simulink model "torque_controller"  (R2018b)
settings: Solver=VariableStepAuto  StartTime=0.0  StopTime=1000  RelTol=1e-3
values from neighbouring files (symbols this model uses):
  ADAMS_cwd = 'C:\Users\Daniel\Documents\GitKraken\DVA439-bicycle-balancing\simulations\simulink'    [Nonlinear_Torque_12km.m]
  ADAMS_exec = ''    [Nonlinear_Torque_12km.m]
  ADAMS_host = 'LAPTOP-BA4FLL9Q'    [Nonlinear_Torque_12km.m]
  ADAMS_init = ''    [Nonlinear_Torque_12km.m]
  ADAMS_inputs = 'TorqueMotor.var_motor_torque!V_In!FrameDisturbance'    [Nonlinear_Torque_12km.m]
  ADAMS_outputs = 'LeanAng_In!SteerAngle!V_Out!Dist!DriftAngle'    [Nonlinear_Torque_12km.m]
  ADAMS_prefix = 'Nonlinear_Torque_12km'    [Nonlinear_Torque_12km.m]
  ADAMS_static = 'no'    [Nonlinear_Torque_12km.m]
  ADAMS_sysdir = 'C:\PROGRA~1\MSC~1.SOF\ADAMSS~1\2018_1\'    [Nonlinear_Torque_12km.m]
libraries: simulink_extras x3, dspsrcs4 x2, simulink x2
settings Model: Creator=Daniel  LastModifiedBy=Daniel
settings SolverCC: AlgebraicLoopSolver=LineSearch

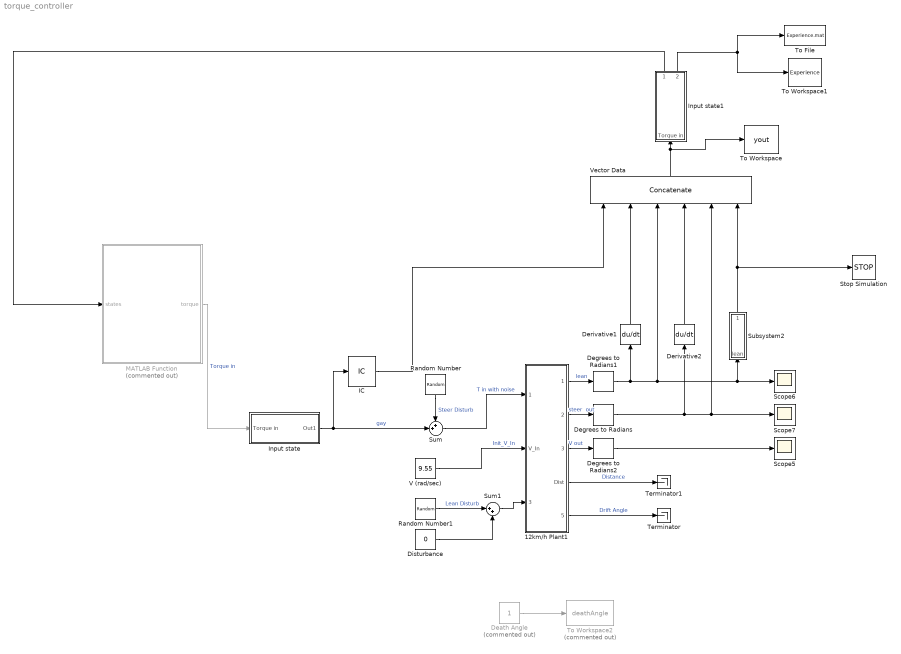
== system torque_controller ==
  12km/h Plant1 : Subsystem
  Death Angle : Constant  Commented=on  SampleTime=-1
  Degrees to Radians : simulink_extras/Transformations/Degrees to Radians
  Degrees to Radians1 : simulink_extras/Transformations/Degrees to Radians
  Degrees to Radians2 : simulink_extras/Transformations/Degrees to Radians
  Derivative1 : Derivative
  Derivative2 : Derivative
  Disturbance : Constant  Value=0
  IC : InitialCondition  Value=0
  Input state : Subsystem
  Input state1 : Subsystem
  MATLAB Function : MATLAB Function  Commented=on  TreatAsAtomicUnit=on
  Random Number : RandomNumber  Variance=0.1  SampleTime=0.1
  Random Number1 : RandomNumber  Variance=0.1  SampleTime=0.1
  Scope5 : Scope
  Scope6 : Scope
  Scope7 : Scope
  Stop Simulation : Stop
  Subsystem2 : Subsystem
  Sum : Sum  Inputs=++|
  Sum1 : Sum  Inputs=|++
  Terminator : Terminator
  Terminator1 : Terminator
  To File : ToFile  Filename=Experience.mat
  To Workspace : ToWorkspace  VariableName=yout  SampleTime=-1
      settings: Save2DSignal=2-D array (concatenate along first dimension)
  To Workspace1 : ToWorkspace  VariableName=Experience  SampleTime=-1
      settings: Decimation=2
  To Workspace2 : ToWorkspace  Commented=on  VariableName=deathAngle  SampleTime=-1
      settings: MaxDataPoints=1
  V (rad/sec) : Constant  Value=9.55
  Vector Data : Concatenate  NumInputs=6
  wires:
  Random Number1/1 -> Sum1/1  "Lean Disturb"
  Disturbance/1 -> Sum1/2
  12km/h Plant1/5(DriftAngle) -> Terminator/1  "Drift Angle"
  Random Number/1 -> Sum/1  "Steer Disturb"
  12km/h Plant1/4("Dist      ") -> Terminator1/1  "Distance"
  Degrees to Radians/1 -> Derivative2/1, Vector Data/5, Scope7/1
  V (rad/sec)/1 -> 12km/h Plant1/2("V_In                        ")  "Init_V_In"
  12km/h Plant1/2(SteerAngle) -> Degrees to Radians/1  "steer  out"
  Sum1/1 -> 12km/h Plant1/3("FrameDisturbance            ")
  12km/h Plant1/3("V_Out     ") -> Degrees to Radians2/1  "V out"
  Sum/1 -> 12km/h Plant1/1(TorqueMotor.var_motor_torque)  "T in with noise"
  Degrees to Radians2/1 -> Scope5/1
  Derivative1/1 -> Vector Data/2
  Derivative2/1 -> Vector Data/4
  Vector Data/1 -> To Workspace/1, Input state1/1(Torque in)
  IC/1 -> Vector Data/1
  Subsystem2/1(dead lean) -> Stop Simulation/1, Vector Data/6
  Death Angle/1 -> To Workspace2/1
  MATLAB Function/1(torque) -> Input state/1(Torque in)  "Torque in"
  Degrees to Radians1/1 -> Derivative1/1, Vector Data/3, Subsystem2/1(lean), Scope6/1
  12km/h Plant1/1(LeanAng_In) -> Degrees to Radians1/1  "lean"
  Input state/1(Out1) -> IC/1, Sum/2  "gay"
  Input state1/1(Out1) -> MATLAB Function/1(states)
  Input state1/2(Out2) -> To File/1, To Workspace1/1

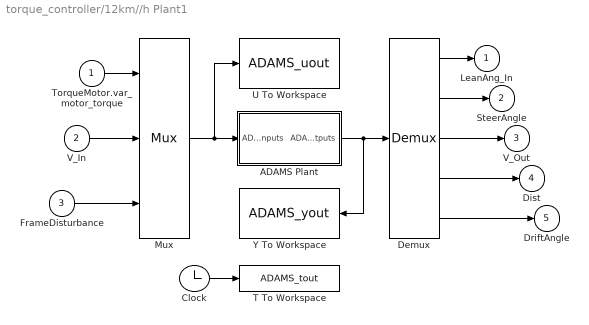
== system torque_controller/12km//h Plant1 ==
  TorqueMotor.var_motor_torque : Inport
  "V_In                        " : Inport  Port=2
  "FrameDisturbance            " : Inport  Port=3
  ADAMS Plant : Subsystem  LoadFcn=|  InitFcn=clear mex  mask(Adams Plant){exevie=ADAMS_sysdir, nam_in=ADAMS_inputs, namout=ADAMS_outputs, nampre=ADAMS_prefix, outfil=ADAMS_prefix, exesol=ADAMS_exec, stat=ADAMS_static, inicmd=[ADAMS_init], exetyp=C++, comtyp=PIPE(DDE), workdir=ADAMS_cwd, ada_host=ADAMS_host, modani=batch, modsim=discrete, dft=no, simulink_lead_cosim=yes, pin_interp_order=0, pout_extrap_order=0, pin_extrap_order=0, pout_interp_order=0, dt_out=0.005, o_rate=1, more=off}
      | %check based on dialog box setting for when setting by popup menu                                             
      | if exist('ADAMS_solver_type')                                                                                 
      |   if strcmp(ADAMS_solver_type,'C++')                                                                          
      |     set_param(gcb,'exetyp','C++');                                                                            
      |   else                                                                                                        
      |     set_param(gcb,'exetyp','Fortran');                                                                        
      |   end                                                                                                         
      | else                                                                                                          
      |   set_param(gcb,'exetyp','C++');                                                                              
      | end                                                                                                           
      | %set the mode if using acar_solver                                                                            
      | %REQUIRED HERE BECAUSE BELOW CAUSES MDLTERMINATE TO BE CALLED 2 TIMES IN MIDDLE OF SIMULATION WHEN SET IN MASK
      |                                                                                                               
      | %enable the direct feedthrough, sim mode, anim mode parameters by default                                     
      |                                                                                                               
      | if exist('set_some_params_states')                                                                            
      |                                                                                                               
      |   set_some_params_states({'dft','modsim','modani'},{'on','on','on'},'MaskEnables',gcb)                        
      |   %turn on direct feedthrough option                                                                          
      |   set_some_params_states({'dft'},{'on'},'MaskVisibilities',gcb)                                               
      |                                                                                                               
      |  end                                                                                                          
      |                                                                                                               
      |                                                                                                               
      | if exist('ADAMS_exec')                                                                                        
      |   if and(strcmp(get_param(gcb,'exesol'),'ADAMS_exec'),strcmp(ADAMS_exec,'acar_solver'))                       
      |     %set the sim mode to discrete -- only supported mode                                                      
      |     set_param(gcb,'modsim','discrete')                                                                        
      |      %turn off direct feedthrough option                                                                      
      |      set_some_params_states({'dft'},{'off'},'MaskVisibilities',gcb)                                           
      |     %set the animation mode to batch -- only supported mode                                                   
      |     set_param(gcb,'modani','batch')                                                                           
      |     %disable the direct feedthrough, sim mode, anim mode parameters                                           
      |     set_some_params_states({'modsim','modani'},{'off','off'},'MaskEnables',gcb)                               
      |   end                                                                                                         
      | end
      mask prompts: exevie "Adams install directory"; nam_in "Adams View input names"; namout "Adams View output names"; nampre "Adams model file prefix"; outfil "Output files prefix (opt.: if blank - no output)"; exesol "User executable (opt.: if blank - use standard)"; stat "Initial static simulation flag"; inicmd "Initialization commands"; exetyp "Adams Solver type"; comtyp "Interprocess option"; workdir "Adams working directory"; ada_host "Adams host"; modani "Animation mode"; modsim "Simulation mode"; dft "Direct feedthrough"; simulink_lead_cosim "Discrete Computational Order - Simulink Leads Adams"; pin_interp_order "Plant input interpolation order"; pout_extrap_order "Plant output extrapolation order"; pin_extrap_order "Plant input extrapolation order"; pout_interp_order "Plant output interpolation order"; dt_out "Communication interval"; o_rate "Number of communications per output step"; more "More parameters"
      mask help: Simulate any Adams plant model either in Adams Solver form (.adm file) or in Adams View form (.cmd file)
      settings: OpenFcn=|
      | open_system(gcb,'mask')
      | if not(exist('set_some_params_states'))
      | 
      | warning('The script "set_some_params_states.m" cannot be found in the MATLAB PATH.  Cannot update the ADAMS Plant S-Function parameters.')
      | 
      | warning('Recommended action(optional):  run the Adams Controls .m file first to help choose the correct settings in the Adams S-Function block.')
      | 
      | end
      mask Help:
      | <html>
      | This S-Function represents the non-linear Adams Plant with the inputs sent to the Adams model <br>
      |  and the outputs generated by the Adams model.  See the Adams Controls documentation for more <br>
      | information.  This plant uses the following variables:<br>
      | <br>
      | <b>ADAMS_sysdir  :</b> Adams installation directory<br>
      | <b>ADAMS_inputs  :</b> Input variables View names vector<br>
      | <b>ADAMS_outputs :</b> Outputs variables View names vector<br>
      | <b>ADAMS_prefix  : </b>ADAMS model files prefix (.adm, .cmd); also doubles as output files prefix<br>
      | <b>ADAMS_exec :</b> Adams Solver user library or keyword (e.g., acar_solver)<br>
      | <b>ADAMS_static :</b> yes|no - initial static before Co-simulation(discrete)/Function Evaluation(continuous)<br>
      | <b>ADAMS_init :</b>Initialization commands (i.e., Adams View or Solver commands, depending on setting for Animation mode)<br>
      | <b>ADAMS_cwd : </b> Current working directory (for TCP/IP)<br>
      | <b>ADAMS_host : </b>Name of Adams server host (for TCP/IP)<br>
      | <b>ADAMS_mode :</b> Linear or non-linear (i.e., co-sim, function eval)<br>
      | <b>ADAMS_solver_type :</b>Fortran or C++ (used to set popup menu when first loaded) <br>
      | 
      | 
      | <br>
      | The following settings can be chosen:<br>
      | <br>
      | <b>Adams Solver type:</b>  Fortran or C++ (will also set ADAMS_solver_type)<br>
      | <b>Interprocess option:</b> Pipe(DDE) or TCP/IP; TCP/IP can allow different machines run Adams and MATLAB<br>
      | <b>Animation mode:</b> batch (Solver, uses .adm) or interactive (View, uses .cmd)<br>
      | <b>Simulation mode:</b> discrete (Co-simulation) or continuous (Function Evaluation)<br>
      | <b>Discrete Computational Order - Simulink Lead Adams:</b> for discrete mode, chooses if Simulink leads the integration (yes) or lags (no);<br> if set to "no", can remove algebraic loop<br>
      | <b>Plant input interpolation order:</b> 0 = zero-order hold; 1 = linear (discrete mode only, where Simulink leads)<br>
      | <b>Plant output extrapolation order:</b> 0 = zero-order hold;1 = linear(discrete mode only, where Simulink leads)<br>
      | <b>Plant input extrapolation order:</b> 0 = zero-order hold; 1 = linear (discrete mode only, where Adams leads)<br>
      | <b>Plant output interpolation order:</b> 0 = zero-order hold;1 = linear(discrete mode only, where Adams leads)<br>
      | <b>Direct feedthrough:</b> yes|no - yes = Input directly effect output(continuous mode-only)<br>
      | <b>Communication interval:</b> Time step at which Co-simulation exchange information (e.g.,0.005); also controls <br>output for continuous mode (Function Evaluation)<br>
      | <b>Number of communications per output step: </b>Sets Adams output rate (.res, .req, .gra) integer value (default: 1)<br>
      | </html>
      mask Callback exesol:
      | if exist('set_some_params_states')
      | %enable the direct feedthrough, sim mode, anim mode parameters
      | set_some_params_states({'dft','modsim','modani'},{'on','on','on'},'MaskEnables',gcb)
      | %turn on direct feedthrough option
      | set_some_params_states({'dft'},{'on'},'MaskVisibilities',gcb)
      | end
      | 
      | if exist('ADAMS_exec')
      |   if and(strcmp(get_param(gcb,'exesol'),'ADAMS_exec'),strcmp(ADAMS_exec,'acar_solver'))
      |     %set the sim mode to discrete -- only supported mode
      |     %REMOVED:  BELOW CAUSES MDLTERMINATE TO BE CALLED 2 TIMES IN MIDDLE OF SIMULATION
      |     %Now in LoadFcn callback
      |     %set_param(gcb,'modsim','discrete')
      |      %turn off direct feedthrough option
      |     set_some_params_states({'dft'},{'off'},'MaskVisibilities',gcb)
      |     %set the animation mode to batch -- only supported mode
      |     %REMOVED:  BELOW CAUSES MDLTERMINATE TO BE CALLED 2 TIMES IN MIDDLE OF SIMULATION
      |     %Now in LoadFcn callback
      |     %set_param(gcb,'modani','batch')
      |     %disable the direct feedthrough, sim mode, anim mode parameters
      |     set_some_params_states({'modsim','modani'},{'off','off'},'MaskEnables',gcb)
      |   end
      | end
      mask TypeOptions exetyp: Fortran | C++
      mask Callback exetyp:
      | if strcmp(get_param(gcb,'exetyp'),'C++')
      |     ADAMS_solver_type='C++';
      | else
      |     ADAMS_solver_type='Fortran';
      | end
      mask TypeOptions comtyp: PIPE(DDE) | TCP/IP
      mask Callback comtyp:
      | if exist('set_some_params_states')
      | if strcmp(get_param(gcb,'comtyp'),'PIPE(DDE)')
      |     %turn off cwd, host options
      |     set_some_params_states({'ada_host','workdir'},{'off','off'},'MaskVisibilities',gcb)
      | else%if strcmp(get_param(gcb,'modsim'),'TCP/IP')
      |     %turn on cwd, host options
      |     set_some_params_states({'ada_host','workdir'},{'on','on'},'MaskVisibilities',gcb)
      | end
      | end
      mask TypeOptions modani: batch | interactive
      mask TypeOptions modsim: discrete | continuous
      mask Callback modsim:
      | if exist('set_some_params_states')
      | if strcmp(get_param(gcb,'modsim'),'discrete')
      |      %turn off direct feedthrough option
      |     set_some_params_states({'dft'},{'off'},'MaskVisibilities',gcb)
      |     %turn on discrete co-sim type if want to see more
      |     if strcmp(get_param(gcb,'more'),'on')
      |         set_some_params_states({'simulink_lead_cosim'},{'on'},'MaskVisibilities',gcb)
      |     end
      |     if strcmp(get_param(gcb,'simulink_lead_cosim'),'yes')
      |         %turn on interpolation/extrapolation options
      |         set_some_params_states({'pin_interp_order','pout_extrap_order',},{'on','on'},'MaskVisibilities',gcb)
      |     else
      |         set_some_params_states({'pin_extrap_order','pout_interp_order'},{'on','on'},'MaskVisibilities',gcb)
      |     end
      | else%if strcmp(get_param(gcb,'modsim'),'continuous')
      |      %turn off direct feedthrough option
      |     set_some_params_states({'dft'},{'on'},'MaskVisibilities',gcb)
      |     %turn off interpolation/extrapolation options
      |     set_some_params_states({'pin_interp_order','pout_extrap_order','pin_extrap_order','pout_interp_order','simulink_lead_cosim'},{'off','off','off','off','off'},'MaskVisibilities',gcb)
      | end
      | end
      mask TypeOptions dft: no | yes
      mask TypeOptions simulink_lead_cosim: yes | no
      mask Callback simulink_lead_cosim:
      | if exist('set_some_params_states')
      | if (strcmp(get_param(gcb,'simulink_lead_cosim'),'yes') && strcmp(get_param(gcb,'modsim'),'discrete'))
      |      %turn off unused interpolate/extrapolate options
      |     set_some_params_states({'pin_extrap_order','pout_interp_order'},{'off','off'},'MaskVisibilities',gcb)
      |     %turn on used interpolate/extrapolate options
      |     set_some_params_states({'pin_interp_order','pout_extrap_order'},{'on','on'},'MaskVisibilities',gcb)
      | elseif (strcmp(get_param(gcb,'simulink_lead_cosim'),'no') && strcmp(get_param(gcb,'modsim'),'discrete'))
      |     %turn on used interpolate/extrapolate options
      |     set_some_params_states({'pin_extrap_order','pout_interp_order'},{'on','on'},'MaskVisibilities',gcb)
      |      %turn off unused interpolate/extrapolate options
      |     set_some_params_states({'pin_interp_order','pout_extrap_order'},{'off','off'},'MaskVisibilities',gcb)
      | end
      | end
      mask TypeOptions pin_interp_order: 0 | 1
      mask TypeOptions pout_extrap_order: 0 | 1
      mask TypeOptions pin_extrap_order: 0 | 1
      mask TypeOptions pout_interp_order: 0 | 1
      mask Callback more:
      | if exist('set_some_params_states')
      | if (strcmp(get_param(gcb,'more'),'on'))
      |      %turn on infrequently used options
      |     set_some_params_states({'exevie','nam_in','namout','exesol','stat','inicmd'},{'on','on','on','on','on','on'},'MaskVisibilities',gcb)
      |     if strcmp(get_param(gcb,'modsim'),'discrete')
      |         set_some_params_states({'simulink_lead_cosim'},{'on'},'MaskVisibilities',gcb)
      |     end
      | elseif (strcmp(get_param(gcb,'more'),'off'))
      |     %turn off infrequently used options
      |     set_some_params_states({'exevie','nam_in','namout','exesol','stat','inicmd'},{'off','off','off','off','off','off'},'MaskVisibilities',gcb)
      |     if strcmp(get_param(gcb,'modsim'),'discrete')
      |         set_some_params_states({'simulink_lead_cosim'},{'off'},'MaskVisibilities',gcb)
      |     end
      | end
      | end
      mask Display: disp( 'MSC Software' )
  Clock : Clock
  Demux : Demux  Outputs=5
  Mux : Mux  Inputs=3
  T To Workspace : ToWorkspace  VariableName=ADAMS_tout
      settings: MaxDataPoints=100000
  U To Workspace : ToWorkspace  VariableName=ADAMS_uout
      settings: MaxDataPoints=100000
  Y To Workspace : ToWorkspace  VariableName=ADAMS_yout
      settings: MaxDataPoints=100000
  LeanAng_In : Outport
  SteerAngle : Outport  Port=2
  "V_Out     " : Outport  Port=3
  "Dist      " : Outport  Port=4
  DriftAngle : Outport  Port=5
  wires:
  "FrameDisturbance            "/1 -> Mux/3
  "V_In                        "/1 -> Mux/2
  TorqueMotor.var_motor_torque/1 -> Mux/1
  Demux/5 -> DriftAngle/1
  Demux/4 -> "Dist      "/1
  Demux/3 -> "V_Out     "/1
  Demux/2 -> SteerAngle/1
  Demux/1 -> LeanAng_In/1
  Mux/1 -> U To Workspace/1, ADAMS Plant/1(ADAMS inputs)
  Clock/1 -> T To Workspace/1
  ADAMS Plant/1(ADAMS outputs) -> Y To Workspace/1, Demux/1

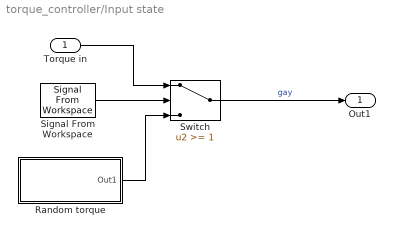
== system torque_controller/Input state ==
  Torque in : Inport
  Random torque : Subsystem
  Signal From Workspace : dspsrcs4/Signal From Workspace  X=torqueState  Ts=1  nsamps=1  OutputAfterFinalValue=Holding final value  ignoreOrWarnInputAndFrameLengths=off  OutputFrames=off
  Switch : Switch  Threshold=1
  Out1 : Outport
  wires:
  Signal From Workspace/1 -> Switch/2
  Random torque/1(Out1) -> Switch/3
  Switch/1 -> Out1/1  "gay"
  Torque in/1 -> Switch/1

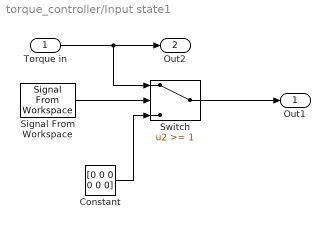
== system torque_controller/Input state1 ==
  Torque in : Inport
  Constant : Constant  Value=[0 0 0 0 0 0]
  Signal From Workspace : dspsrcs4/Signal From Workspace  X=torqueState  Ts=1  nsamps=1  OutputAfterFinalValue=Holding final value  ignoreOrWarnInputAndFrameLengths=off  OutputFrames=off
  Switch : Switch  Threshold=1
  Out1 : Outport
  Out2 : Outport  Port=2
  wires:
  Signal From Workspace/1 -> Switch/2
  Torque in/1 -> Out2/1, Switch/1
  Constant/1 -> Switch/3
  Switch/1 -> Out1/1

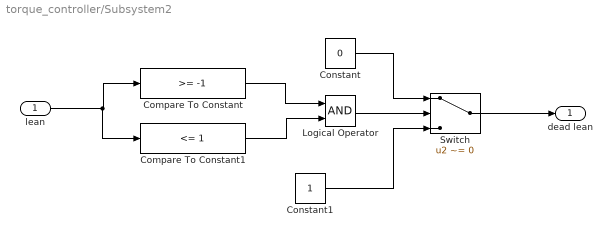
== system torque_controller/Subsystem2 ==
  lean : Inport
  Compare To Constant : simulink/Logic and Bit Operations/Compare To Constant  relop=>=  const=-1  OutDataTypeStr=boolean
  Compare To Constant1 : simulink/Logic and Bit Operations/Compare To Constant  relop=<=  const=1  OutDataTypeStr=boolean
  Constant : Constant  Value=0
  Constant1 : Constant
  Logical Operator : Logic  AllPortsSameDT=off  OutDataTypeStr=boolean
  Switch : Switch  Criteria=u2 ~= 0
  dead lean : Outport
  wires:
  Switch/1 -> dead lean/1
  Compare To Constant1/1 -> Logical Operator/2
  lean/1 -> Compare To Constant1/1, Compare To Constant/1
  Logical Operator/1 -> Switch/2
  Compare To Constant/1 -> Logical Operator/1
  Constant/1 -> Switch/1
  Constant1/1 -> Switch/3

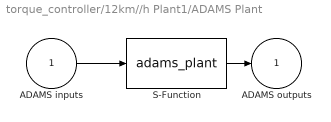
== system torque_controller/12km//h Plant1/ADAMS Plant ==
  ADAMS inputs : Inport
  S-Function : S-Function  StopFcn=clear mex  FunctionName=adams_plant  Parameters=exevie,exesol,stat,outfil,nampre,o_rate,nam_in,namout,dft,modsim,modani,dt_out,inicmd,exetyp,comtyp,ada_host, workdir,pin_interp_order,pout_extrap_order,pin_extrap_order,pout_interp_order,simulink_lead_cosim  SFunctionDeploymentMode=off  EnableBusSupport=off
  ADAMS outputs : Outport  InitialOutput=0
  wires:
  S-Function/1 -> ADAMS outputs/1
  ADAMS inputs/1 -> S-Function/1

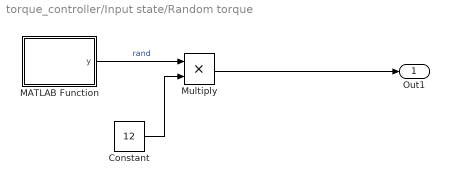
== system torque_controller/Input state/Random torque ==
  Constant : Constant  Value=12
  MATLAB Function : MATLAB Function  TreatAsAtomicUnit=on
  Multiply : Product
  Out1 : Outport
  wires:
  MATLAB Function/1(y) -> Multiply/1  "rand"
  Constant/1 -> Multiply/2
  Multiply/1 -> Out1/1

== matlab function torque_controller/Input state/Random torque/MATLAB Function ==
  data: y output
function y = fcn
%#codegen
coder.extrinsic('rand','rng');
y = 0;

persistent atTime0
if isempty(atTime0)
    rng('shuffle');
    atTime0 = false;
end

y = rand;

y = round(y);

if (y==0)
    y = -1;
end

== matlab function torque_controller/MATLAB Function ==
  data: states input; torque output
function torque  = kit(states)

previousTorque = states(:,1);
deriv_leanAngle = states(:,2);
leanAngle = states(:,3);
steerAngle = states(:,4);
deriv_steerAngle = states(:,5);
death_state = states(:,6);

%%%%%%%%%%%%%%%%%%%%%%%%%%%%%%%%%%%%%%%%%%%%%%%%%%%%%%%%%%%%%%%%%%%%%%%%%%%%%%%%%%%%%
% Setup initial experiences
%%%%%%%%%%%%%%%%%%%%%%%%%%%%%%%%%%%%%%%%%%%%%%%%%%%%%%%%%%%%%%%%%%%%%%%%%%%%%%%%%%%%%
TrSet = {};
Input = [];

currentState = states;
% State array
TrSet{1, i} = [currentState];
% Action array
% First index in the action array is never used but needed due to size issues when expanding the episode
TrSet{2, i} = [0];

while(abs(currentState(1)) <= deathCartPos && abs(currentState(3))<=deathPoleAngle)
    action = actions(floor(4*rand)+1);
    nextState = SimulatePendel(action*(1 + 0.2*(2*rand - 1)), currentState(1), currentState(2), currentState(3), currentState(4));
    TrSet{1, i} = [TrSet{1, i} ; nextState];
    TrSet{2, i} = [TrSet{2, i}; action];
    currentState = nextState;
end
% Calculate the costs of the future state, use 0.1/0.9 instead of 0/1 to accomodate sigmoid function.
Target = 0.10 + 0.80*(abs(TrSet{1,i}(:,3)) > allowedPoleAngle | abs(TrSet{1,i}(:,1)) > allowedCartPos);
% Recursivly expand the 'input' cell array with 'state, action, cost' - tripplets
Input = [Input; TrSet{1,i}(1:end-1,:) TrSet{2,i}(2:end,:) Target(2:end)];

%%%%%%%%%%%%%%%%%%%%%%%%%%%%%%%%%%%%%%%%%%%%%%%%%%%%%%%%%%%%%%%%%%%%%%%%%%%%%%%%%%%%%
% Initiate network
% Random weight/bias initiation
% Training fuction can be set inside initNN()
%%%%%%%%%%%%%%%%%%%%%%%%%%%%%%%%%%%%%%%%%%%%%%%%%%%%%%%%%%%%%%%%%%%%%%%%%%%%%%%%%%%%%
net = initNN(Input(:,1:5)', Input(:,6)', [10 10]);

%%%%%%%%%%%%%%%%%%%%%%%%%%%%%%%%%%%%%%%%%%%%%%%%%%%%%%%%%%%%%%%%%%%%%%%%%%%%%%%%%%%%%
% Q-fitted training
%%%%%%%%%%%%%%%%%%%%%%%%%%%%%%%%%%%%%%%%%%%%%%%%%%%%%%%%%%%%%%%%%%%%%%%%%%%%%%%%%%%%%

% Used to indicate savepoints of network 
bestActionNr = 0;
% Goal of the training
maxRange = 1000;
for k = 1:12
    for i = 1:100
        currentState = startState;
        TrSet{1, i} = [currentState];
        TrSet{2, i} = [0];
        actionNr = 0;

        while(abs(currentState(1)) <= deathCartPos && abs(currentState(3))<=deathPoleAngle && actionNr < maxRange)

            % Exploration 1/(epsilon) of the time, set false if no exploration
            epsilon = 1+k;
            if(mod(actionNr, epsilon) == 0 && true)
                action = actions(floor(4*rand)+1);
            else
                Q1 = net([currentState actions(1)]');
                Q2 = net([currentState actions(2)]');
                Q3 = net([currentState actions(3)]');
                Q4 = net([currentState actions(4)]');

                [mv, index] = min([Q1 Q2 Q3 Q4]);
                action = actions(index);
            end
            %Next state is suspect to a random noise with magnitude 20% of action '*(1 + 0.2*(2*rand - 1))'
            nextState = SimulatePendel(action, currentState(1), currentState(2), currentState(3), currentState(4));
            TrSet{1, i} = [TrSet{1, i} ; nextState];
            TrSet{2, i} = [TrSet{2, i}; action];
            currentState = nextState;
            actionNr = actionNr + 1;

            %Set display of internal loop on
            clc;
            if (true)
                disp('Episode: ');
                disp(i);
                disp('Survival Actions: ');
                disp(actionNr);
                disp('Best Survival Actions: ')
                disp(bestActionNr)
            end
            %Set display of external loop on
            if (true)
                disp('Training Iteration: ')
                disp(k-1) 
            end
        end

        %Save best net
        if actionNr > bestActionNr
            bestNet = net;
            bestActionNr = actionNr;
        end

        % Calculate cost of next state
        Target = 0.05 + 0.90*(abs(TrSet{1,i}(:,3)) > allowedPoleAngle | abs(TrSet{1,i}(:,1)) > allowedCartPos);
        Input = [Input; [TrSet{1,i}(1:end-1,:) TrSet{2,i}(2:end,:)] Target(2:end)];

    end
    [net,tr] = train(net,Input(:,1:5)', Input(:,6)');
end
net = bestNet;
